simulink model "Simulator_Template_FreeFlight"  (Simulink 8.1)
settings: Solver=ode45  StartTime=0.0  StopTime=10.0  RelTol=1e-3
values from neighbouring files (symbols this model uses):
  g = 9.8065    [kostas_malakies.mat]    (also in kostas_malakies2.mat; load_PMModel.m = 9.81; main.m; main_last.m)
  mass = 0.66    [kostas_malakies.mat]    (also in kostas_malakies2.mat; load_PMModel.m = 0.687; main_last.m)
  z = [-0.93079906702 -0.933865725994 -0.937557637691 -0.939011216164 -0.94143640995 -0.944628417492 -0.947235524654 -0.949601888657 -0.952827751637 -0.9567258358 -0.958320975304 -0.960991024971 ... (7988 elements, 7988x1)]    [kostas_malakies2.mat]    (also in plotDataTest.m = simout_data.signals.values(:,11))
libraries: Hquad_control_LIB_MPC x2, Hqaud_model_LIB_SI x1
settings Model: Creator=root  LastModifiedBy=root
settings DataIOCC: SignalLoggingSaveFormat=Dataset
settings OptimizationCC: ExpressionDepthLimit=128
settings DebuggingCC: FcnCallInpInsideContextMsg=EnableAllAsError
settings GRTTargetCC: CombineOutputUpdateFcns=on  GRTInterface=off

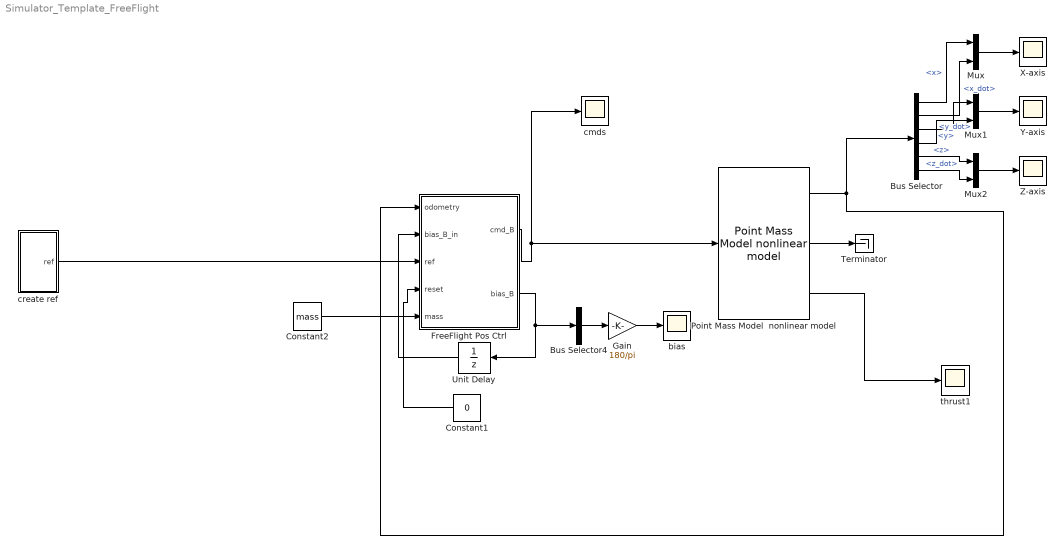
== system Simulator_Template_FreeFlight ==
  Bus Selector : BusSelector  OutputSignals=pos.x,vel.x_dot,pos.y,vel.y_dot,pos.z,vel.z_dot
  Bus Selector4 : BusSelector  OutputSignals=pitch_bias,roll_bias,thrust_bias  OutputAsBus=on
  Constant1 : Constant  Value=0
  Constant2 : Constant  Value=mass
  FreeFlight Pos Ctrl : Subsystem  AncestorBlock=Hquad_control_LIB_MPC/pos controller
  Gain : Gain  Gain=180/pi
  Mux : Mux  Inputs=2
  Mux1 : Mux  Inputs=2
  Mux2 : Mux  Inputs=2
  Point Mass Model  nonlinear model : Hqaud_model_LIB_SI/Point Mass Model  nonlinear model
  Terminator : Terminator
  Unit Delay : UnitDelay  SampleTime=-1
  X-axis : Scope
      settings: TimeRange=40  YMin=-0.5  YMax=0.5  SaveName=ScopeData3
  Y-axis : Scope
      settings: TimeRange=40  YMin=-0.5  YMax=0.5  SaveName=ScopeData4
  Z-axis : Scope
      settings: TimeRange=40  YMin=-0.5  YMax=0.5  SaveName=ScopeData5
  bias : Scope
      settings: TimeRange=39.996  YMin=-0.07  YMax=0.05
  cmds : Scope
      settings: TimeRange=40  YMin=-0.5  YMax=0.5
  create ref : Subsystem  AncestorBlock=Hquad_control_LIB_LQRI/create ref
  thrust1 : Scope
      settings: TimeRange=40  YMin=-2  YMax=6  SaveName=ScopeData6
  wires:
  Point Mass Model  nonlinear model/2 -> Terminator/1
  Constant1/1 -> FreeFlight Pos Ctrl/4(reset)
  Point Mass Model  nonlinear model/1 -> FreeFlight Pos Ctrl/1(odometry), Bus Selector/1
  FreeFlight Pos Ctrl/1(cmd_B) -> Point Mass Model  nonlinear model/1, cmds/1
  FreeFlight Pos Ctrl/2(bias_B) -> Unit Delay/1, Bus Selector4/1
  Bus Selector4/1 -> Gain/1
  Gain/1 -> bias/1
  Unit Delay/1 -> FreeFlight Pos Ctrl/2(bias_B_in)
  Constant2/1 -> FreeFlight Pos Ctrl/5(mass)
  create ref/1(ref) -> FreeFlight Pos Ctrl/3(ref)
  Point Mass Model  nonlinear model/3 -> thrust1/1
  Mux/1 -> X-axis/1
  Bus Selector/1 -> Mux/1  "<x>"
  Bus Selector/2 -> Mux/2  "<x_dot>"
  Bus Selector/3 -> Mux1/1  "<y>"
  Bus Selector/4 -> Mux1/2  "<y_dot>"
  Bus Selector/5 -> Mux2/1  "<z>"
  Bus Selector/6 -> Mux2/2  "<z_dot>"
  Mux1/1 -> Y-axis/1
  Mux2/1 -> Z-axis/1

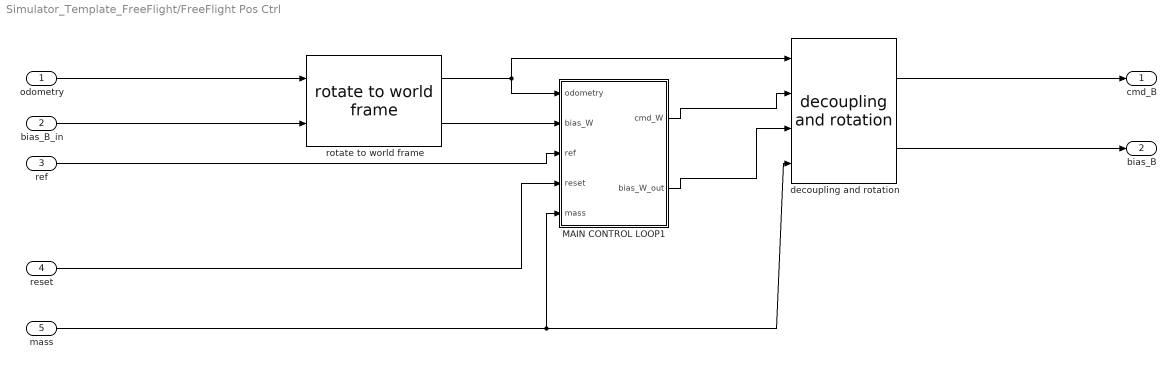
== system Simulator_Template_FreeFlight/FreeFlight Pos Ctrl ==
  odometry : Inport
  bias_B_in : Inport  Port=2
  ref : Inport  Port=3
  reset : Inport  Port=4
  mass : Inport  Port=5
  MAIN CONTROL LOOP1 : Subsystem  Priority=2  AncestorBlock=Hquad_control_LIB_MPC/MAIN CONTROL LOOP  TreatAsAtomicUnit=on
  decoupling and rotation : Hquad_control_LIB_MPC/decoupling and rotation  Priority=3
  rotate to world frame : Hquad_control_LIB_MPC/rotate to world frame  Priority=1
  cmd_B : Outport
  bias_B : Outport  Port=2
  wires:
  mass/1 -> decoupling and rotation/4, MAIN CONTROL LOOP1/5(mass)
  bias_B_in/1 -> rotate to world frame/2
  rotate to world frame/2 -> MAIN CONTROL LOOP1/2(bias_W)
  decoupling and rotation/2 -> bias_B/1
  decoupling and rotation/1 -> cmd_B/1
  MAIN CONTROL LOOP1/2(bias_W_out) -> decoupling and rotation/3
  rotate to world frame/1 -> decoupling and rotation/1, MAIN CONTROL LOOP1/1(odometry)
  ref/1 -> MAIN CONTROL LOOP1/3(ref)
  reset/1 -> MAIN CONTROL LOOP1/4(reset)
  MAIN CONTROL LOOP1/1(cmd_W) -> decoupling and rotation/2
  odometry/1 -> rotate to world frame/1

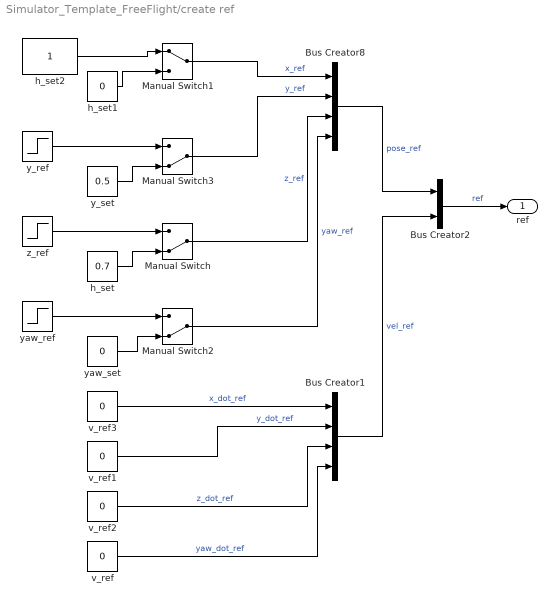
== system Simulator_Template_FreeFlight/create ref ==
  Bus Creator1 : BusCreator
  Bus Creator2 : BusCreator  Inputs=2
  Bus Creator8 : BusCreator
  Manual Switch : ManualSwitch  CurrentSetting=0
  Manual Switch1 : ManualSwitch
  Manual Switch2 : ManualSwitch  CurrentSetting=0
  Manual Switch3 : ManualSwitch  CurrentSetting=0
  h_set : Constant  Value=0.7  OutDataTypeStr=double  SampleTime=-1
  h_set1 : Constant  Value=0  OutDataTypeStr=double  SampleTime=-1
  h_set2 : Constant  OutDataTypeStr=double  SampleTime=-1
  v_ref{,1..3} (4 alike) : Constant  Value=0  OutDataTypeStr=double  SampleTime=-1
  y_ref : Step  Time=15  SampleTime=0
  y_set : Constant  Value=0.5  OutDataTypeStr=double  SampleTime=-1
  yaw_ref : Step  Time=20  After=pi  SampleTime=0
  "yaw_set  " : Constant  Value=0  OutDataTypeStr=double  SampleTime=-1
  z_ref : Step  Time=15  SampleTime=0
  ref : Outport
  wires:
  h_set2/1 -> Manual Switch1/1
  v_ref2/1 -> Bus Creator1/3  "z_dot_ref"
  v_ref1/1 -> Bus Creator1/2  "y_dot_ref"
  v_ref3/1 -> Bus Creator1/1  "x_dot_ref"
  v_ref/1 -> Bus Creator1/4  "yaw_dot_ref"
  Manual Switch/1 -> Bus Creator8/3  "z_ref"
  Manual Switch2/1 -> Bus Creator8/4  "yaw_ref"
  Manual Switch3/1 -> Bus Creator8/2  "y_ref"
  Manual Switch1/1 -> Bus Creator8/1  "x_ref"
  Bus Creator1/1 -> Bus Creator2/2  "vel_ref"
  Bus Creator8/1 -> Bus Creator2/1  "pose_ref"
  Bus Creator2/1 -> ref/1  "ref"
  h_set1/1 -> Manual Switch1/2
  y_set/1 -> Manual Switch3/2
  y_ref/1 -> Manual Switch3/1
  z_ref/1 -> Manual Switch/1
  h_set/1 -> Manual Switch/2
  "yaw_set  "/1 -> Manual Switch2/2
  yaw_ref/1 -> Manual Switch2/1

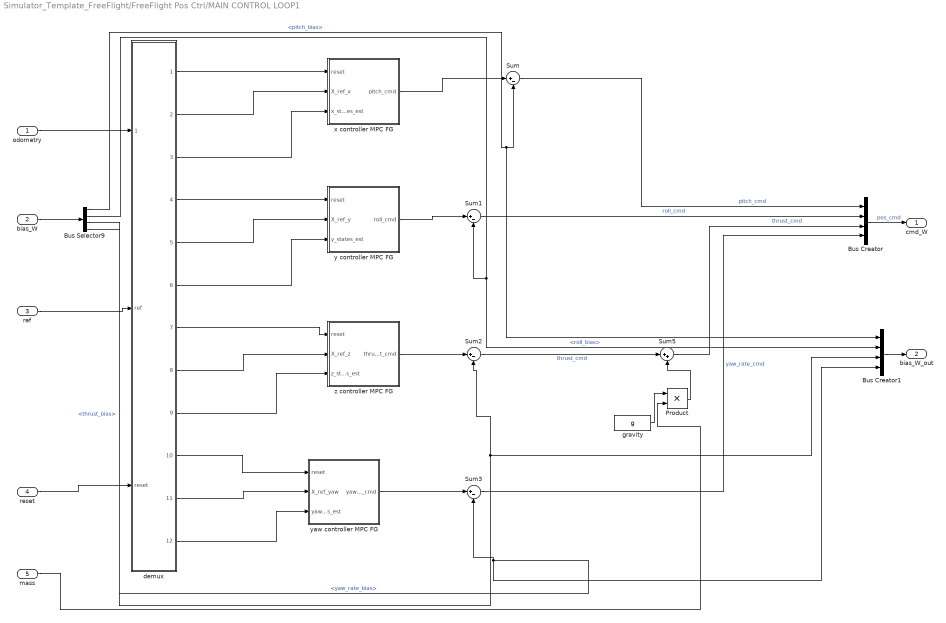
== system Simulator_Template_FreeFlight/FreeFlight Pos Ctrl/MAIN CONTROL LOOP1 ==
  odometry : Inport
  bias_W : Inport  Port=2
  ref : Inport  Port=3
  reset : Inport  Port=4
  mass : Inport  Port=5
  Bus Creator : BusCreator
  Bus Creator1 : BusCreator
  Bus Selector9 : BusSelector  OutputSignals=pitch_bias,roll_bias,thrust_bias,yaw_rate_bias
  Product : Product  RndMeth=Zero
  Sum{,1..3} (4 alike) : Sum  Inputs=|+-
  Sum5 : Sum  Inputs=|++
  demux : Subsystem
  gravity : Constant  Value=g
  "x controller MPC FG  " : Subsystem  AncestorBlock=Hquad_control_LIB_MPC/x controller MPC FG
  y controller MPC FG : Subsystem  AncestorBlock=Hquad_control_LIB_MPC/y controller MPC FG
  yaw controller MPC FG : Subsystem  AncestorBlock=Hquad_control_LIB_MPC/yaw controller MPC FG
  z controller MPC FG : Subsystem  AncestorBlock=Hquad_control_LIB_MPC/z controller MPC FG
  cmd_W : Outport
  bias_W_out : Outport  Port=2
  wires:
  Bus Selector9/4 -> Sum3/2, Bus Creator1/4  "<yaw_rate_bias>"
  Sum3/1 -> Bus Creator/4  "yaw_rate_cmd"
  Bus Selector9/3 -> Sum2/2, Bus Creator1/3  "<thrust_bias>"
  Bus Selector9/1 -> Sum/2, Bus Creator1/1  "<pitch_bias>"
  Bus Selector9/2 -> Bus Creator1/2, Sum1/2  "<roll_bias>"
  bias_W/1 -> Bus Selector9/1
  Sum5/1 -> Bus Creator/3  "thrust_cmd"
  Bus Creator1/1 -> bias_W_out/1
  Sum2/1 -> Sum5/1  "thrust_cmd"
  Sum1/1 -> Bus Creator/2  "roll_cmd"
  Sum/1 -> Bus Creator/1  "pitch_cmd"
  odometry/1 -> demux/1(odometry)
  ref/1 -> demux/2(ref)
  reset/1 -> demux/3(reset)
  demux/1(reset1) -> "x controller MPC FG  "/1(reset)
  demux/4(reset2) -> y controller MPC FG/1(reset)
  demux/7(reset3) -> z controller MPC FG/1(reset)
  demux/10(reset4) -> yaw controller MPC FG/1(reset)
  Bus Creator/1 -> cmd_W/1  "pos_cmd"
  mass/1 -> Product/2
  Product/1 -> Sum5/2
  gravity/1 -> Product/1
  "x controller MPC FG  "/1("pitch_cmd   ") -> Sum/1
  y controller MPC FG/1(roll_cmd) -> Sum1/1
  z controller MPC FG/1(thrust_cmd) -> Sum2/1
  yaw controller MPC FG/1(yaw_rate_cmd) -> Sum3/1
  demux/2(X_ref_x) -> "x controller MPC FG  "/2("X_ref_x  ")
  demux/3(x_states) -> "x controller MPC FG  "/3("x_states_est  ")
  demux/5(X_ref_y) -> y controller MPC FG/2("X_ref_y  ")
  demux/6(y_states) -> y controller MPC FG/3("y_states_est  ")
  demux/8(X_ref_z) -> z controller MPC FG/2(X_ref_z)
  demux/9(z_states) -> z controller MPC FG/3("z_states_est  ")
  demux/11(X_ref_yaw) -> yaw controller MPC FG/2(X_ref_yaw)
  demux/12(yaw_states) -> yaw controller MPC FG/3("yaw_states_est  ")

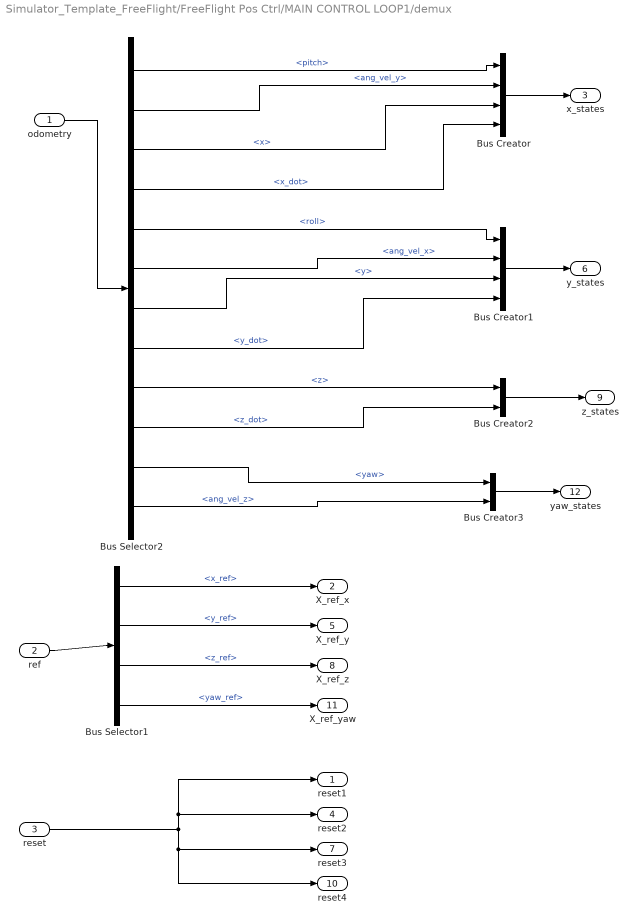
== system Simulator_Template_FreeFlight/FreeFlight Pos Ctrl/MAIN CONTROL LOOP1/demux ==
  odometry : Inport
  ref : Inport  Port=2
  reset : Inport  Port=3
  Bus Creator : BusCreator
  Bus Creator1 : BusCreator
  Bus Creator2 : BusCreator  Inputs=2
  Bus Creator3 : BusCreator  Inputs=2
  Bus Selector1 : BusSelector  OutputSignals=pose_ref.x_ref,pose_ref.y_ref,pose_ref.z_ref,pose_ref.yaw_ref
  Bus Selector2 : BusSelector  OutputSignals=rpy.pitch,ang_vel.ang_vel_y,pos.x,vel.x_dot,rpy.roll,ang_vel.ang_vel_x,pos.y,vel.y_dot,pos.z,vel.z_dot,rpy.yaw,ang_vel.ang_vel_z
  reset1 : Outport
  X_ref_x : Outport  Port=2
  x_states : Outport  Port=3
  reset2 : Outport  Port=4
  X_ref_y : Outport  Port=5
  y_states : Outport  Port=6
  reset3 : Outport  Port=7
  X_ref_z : Outport  Port=8
  z_states : Outport  Port=9
  reset4 : Outport  Port=10
  X_ref_yaw : Outport  Port=11
  yaw_states : Outport  Port=12
  wires:
  Bus Selector1/4 -> X_ref_yaw/1  "<yaw_ref>"
  Bus Selector1/3 -> X_ref_z/1  "<z_ref>"
  odometry/1 -> Bus Selector2/1
  ref/1 -> Bus Selector1/1
  Bus Selector1/1 -> X_ref_x/1  "<x_ref>"
  Bus Selector1/2 -> X_ref_y/1  "<y_ref>"
  reset/1 -> reset3/1, reset4/1, reset2/1, reset1/1
  Bus Creator/1 -> x_states/1
  Bus Selector2/1 -> Bus Creator/1  "<pitch>"
  Bus Selector2/2 -> Bus Creator/2  "<ang_vel_y>"
  Bus Selector2/3 -> Bus Creator/3  "<x>"
  Bus Selector2/4 -> Bus Creator/4  "<x_dot>"
  Bus Creator1/1 -> y_states/1
  Bus Selector2/5 -> Bus Creator1/1  "<roll>"
  Bus Selector2/6 -> Bus Creator1/2  "<ang_vel_x>"
  Bus Selector2/7 -> Bus Creator1/3  "<y>"
  Bus Selector2/8 -> Bus Creator1/4  "<y_dot>"
  Bus Selector2/9 -> Bus Creator2/1  "<z>"
  Bus Selector2/10 -> Bus Creator2/2  "<z_dot>"
  Bus Selector2/12 -> Bus Creator3/2  "<ang_vel_z>"
  Bus Selector2/11 -> Bus Creator3/1  "<yaw>"
  Bus Creator2/1 -> z_states/1
  Bus Creator3/1 -> yaw_states/1

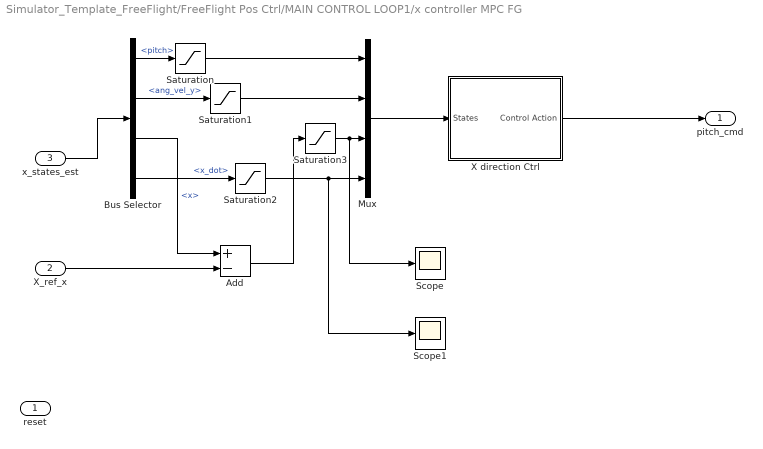
== system Simulator_Template_FreeFlight/FreeFlight Pos Ctrl/MAIN CONTROL LOOP1/x controller MPC FG   ==
  reset : Inport  PortDimensions=1
  "X_ref_x  " : Inport  Port=2
  "x_states_est  " : Inport  Port=3
  Add : Sum  Inputs=+-
  Bus Selector : BusSelector  OutputSignals=pitch,ang_vel_y,x,x_dot
  Mux : Mux
  Saturation : Saturate  UpperLimit=0.2094  LowerLimit=-0.2094
  Saturation1 : Saturate  UpperLimit=2  LowerLimit=-2
  Saturation2 : Saturate  UpperLimit=1  LowerLimit=-1
  Saturation3 : Saturate  UpperLimit=1  LowerLimit=-1
  Scope : Scope
      settings: SaveName=ScopeData11
  Scope1 : Scope
      settings: SaveName=ScopeData12
  X direction Ctrl : Subsystem  AncestorBlock=mpt_sim/Explicit Controller  mask(MPT Controller){}
      mask help: Evaluates explicit controller for a given state.
      mask Help: Evaluation of an explicit control law is performed by the C-code S-function "mpt_getInput_sfunc", which requires the controller to be exported to C-code using "exportToC".
      mask Display: image(imread('mpt_ctrl.jpg'));
  "pitch_cmd   " : Outport  PortDimensions=1
  wires:
  X direction Ctrl/1(Control Action) -> "pitch_cmd   "/1
  "X_ref_x  "/1 -> Add/2
  Bus Selector/1 -> Saturation/1  "<pitch>"
  Bus Selector/2 -> Saturation1/1  "<ang_vel_y>"
  Bus Selector/3 -> Add/1  "<x>"
  Add/1 -> Saturation3/1
  Bus Selector/4 -> Saturation2/1  "<x_dot>"
  Mux/1 -> X direction Ctrl/1(States)
  "x_states_est  "/1 -> Bus Selector/1
  Saturation/1 -> Mux/1
  Saturation1/1 -> Mux/2
  Saturation2/1 -> Scope1/1, Mux/4
  Saturation3/1 -> Scope/1, Mux/3

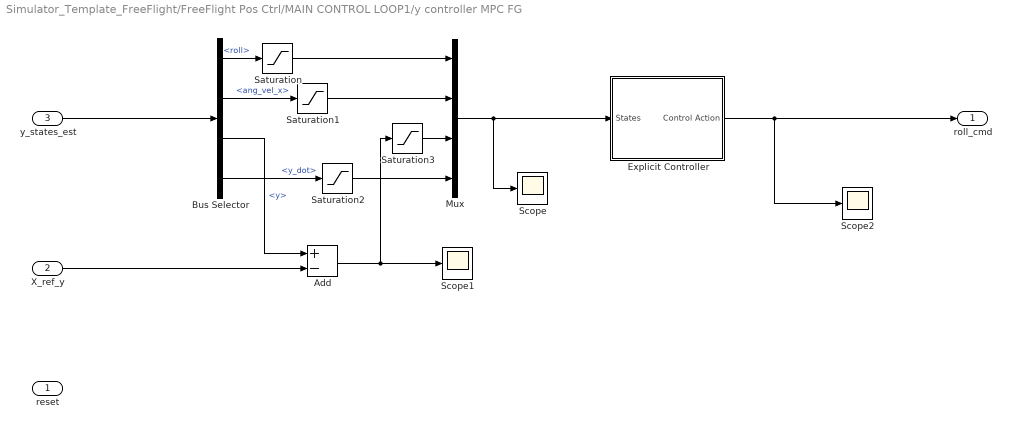
== system Simulator_Template_FreeFlight/FreeFlight Pos Ctrl/MAIN CONTROL LOOP1/y controller MPC FG ==
  reset : Inport  PortDimensions=1
  "X_ref_y  " : Inport  Port=2
  "y_states_est  " : Inport  Port=3
  Add : Sum  Inputs=+-
  Bus Selector : BusSelector  OutputSignals=roll,ang_vel_x,y,y_dot
  Explicit Controller : Subsystem  AncestorBlock=mpt_sim/Explicit Controller  mask(MPT Controller){}
      mask help: Evaluates explicit controller for a given state.
      mask Help: Evaluation of an explicit control law is performed by the C-code S-function "mpt_getInput_sfunc", which requires the controller to be exported to C-code using "exportToC".
      mask Display: image(imread('mpt_ctrl.jpg'));
  Mux : Mux
  Saturation : Saturate  UpperLimit=0.2094  LowerLimit=-0.2094
  Saturation1 : Saturate  UpperLimit=2  LowerLimit=-2
  Saturation2 : Saturate  UpperLimit=1  LowerLimit=-1
  Saturation3 : Saturate  UpperLimit=1  LowerLimit=-1
  Scope : Scope
      settings: SaveName=ScopeData3
  Scope1 : Scope
      settings: SaveName=ScopeData5
  Scope2 : Scope
      settings: SaveName=ScopeData6
  roll_cmd : Outport  PortDimensions=1
  wires:
  Explicit Controller/1(Control Action) -> Scope2/1, roll_cmd/1
  "X_ref_y  "/1 -> Add/2
  Bus Selector/1 -> Saturation/1  "<roll>"
  Bus Selector/2 -> Saturation1/1  "<ang_vel_x>"
  Bus Selector/3 -> Add/1  "<y>"
  Add/1 -> Scope1/1, Saturation3/1
  Bus Selector/4 -> Saturation2/1  "<y_dot>"
  Mux/1 -> Scope/1, Explicit Controller/1(States)
  "y_states_est  "/1 -> Bus Selector/1
  Saturation/1 -> Mux/1
  Saturation1/1 -> Mux/2
  Saturation2/1 -> Mux/4
  Saturation3/1 -> Mux/3

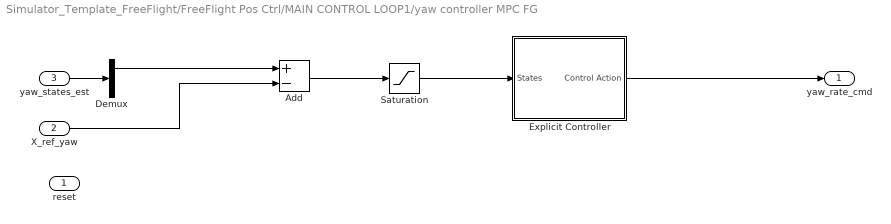
== system Simulator_Template_FreeFlight/FreeFlight Pos Ctrl/MAIN CONTROL LOOP1/yaw controller MPC FG ==
  reset : Inport  PortDimensions=1
  X_ref_yaw : Inport  Port=2
  "yaw_states_est  " : Inport  Port=3
  Add : Sum  Inputs=+-
  Demux : Demux  Outputs=2
  Explicit Controller : Subsystem  AncestorBlock=mpt_sim/Explicit Controller  mask(MPT Controller){}
      mask help: Evaluates explicit controller for a given state.
      mask Help: Evaluation of an explicit control law is performed by the C-code S-function "mpt_getInput_sfunc", which requires the controller to be exported to C-code using "exportToC".
      mask Display: image(imread('mpt_ctrl.jpg'));
  Saturation : Saturate  UpperLimit=0.0873  LowerLimit=-0.0873
  yaw_rate_cmd : Outport  PortDimensions=1
  wires:
  X_ref_yaw/1 -> Add/2
  "yaw_states_est  "/1 -> Demux/1
  Demux/1 -> Add/1
  Add/1 -> Saturation/1
  Explicit Controller/1(Control Action) -> yaw_rate_cmd/1
  Saturation/1 -> Explicit Controller/1(States)

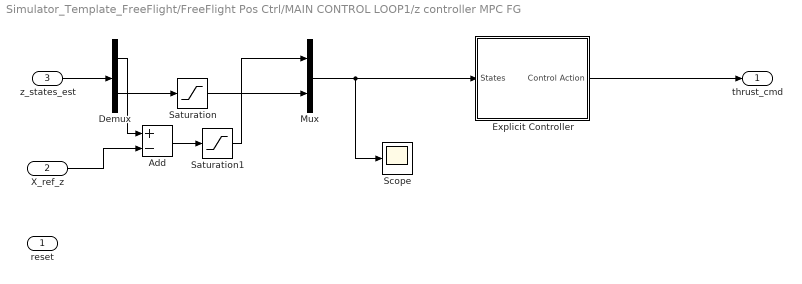
== system Simulator_Template_FreeFlight/FreeFlight Pos Ctrl/MAIN CONTROL LOOP1/z controller MPC FG ==
  reset : Inport  PortDimensions=1
  X_ref_z : Inport  Port=2
  "z_states_est  " : Inport  Port=3
  Add : Sum  Inputs=+-
  Demux : Demux  Outputs=2
  Explicit Controller : Subsystem  AncestorBlock=mpt_sim/Explicit Controller  mask(MPT Controller){}
      mask help: Evaluates explicit controller for a given state.
      mask Help: Evaluation of an explicit control law is performed by the C-code S-function "mpt_getInput_sfunc", which requires the controller to be exported to C-code using "exportToC".
      mask Display: image(imread('mpt_ctrl.jpg'));
  Mux : Mux  Inputs=2
  Saturation : Saturate  UpperLimit=1  LowerLimit=-1
  Saturation1 : Saturate  UpperLimit=1  LowerLimit=-1
  Scope : Scope
      settings: SaveName=ScopeData2
  thrust_cmd : Outport  PortDimensions=1
  wires:
  "z_states_est  "/1 -> Demux/1
  Demux/2 -> Saturation/1
  Demux/1 -> Add/1
  X_ref_z/1 -> Add/2
  Add/1 -> Saturation1/1
  Explicit Controller/1(Control Action) -> thrust_cmd/1
  Mux/1 -> Scope/1, Explicit Controller/1(States)
  Saturation/1 -> Mux/2
  Saturation1/1 -> Mux/1

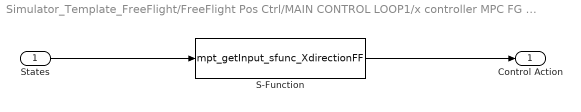
== system Simulator_Template_FreeFlight/FreeFlight Pos Ctrl/MAIN CONTROL LOOP1/x controller MPC FG  /X direction Ctrl ==
  States : Inport
  S-Function : S-Function  FunctionName=mpt_getInput_sfunc_XdirectionFF  EnableBusSupport=off
  Control Action : Outport
  wires:
  S-Function/1 -> Control Action/1
  States/1 -> S-Function/1

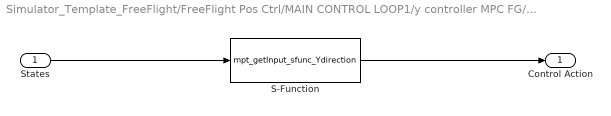
== system Simulator_Template_FreeFlight/FreeFlight Pos Ctrl/MAIN CONTROL LOOP1/y controller MPC FG/Explicit Controller ==
  States : Inport
  S-Function : S-Function  FunctionName=mpt_getInput_sfunc_Ydirection  EnableBusSupport=off
  Control Action : Outport
  wires:
  S-Function/1 -> Control Action/1
  States/1 -> S-Function/1

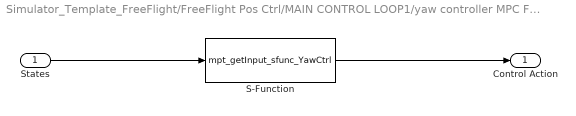
== system Simulator_Template_FreeFlight/FreeFlight Pos Ctrl/MAIN CONTROL LOOP1/yaw controller MPC FG/Explicit Controller ==
  States : Inport
  S-Function : S-Function  FunctionName=mpt_getInput_sfunc_YawCtrl  EnableBusSupport=off
  Control Action : Outport
  wires:
  S-Function/1 -> Control Action/1
  States/1 -> S-Function/1

== system Simulator_Template_FreeFlight/FreeFlight Pos Ctrl/MAIN CONTROL LOOP1/z controller MPC FG/Explicit Controller ==
  States : Inport
  S-Function : S-Function  FunctionName=mpt_getInput_sfunc_Zdirection  EnableBusSupport=off
  Control Action : Outport
  wires:
  S-Function/1 -> Control Action/1
  States/1 -> S-Function/1
